simulink model "TestCollecteurAdmissionNew"  (R2024b)
settings: Solver=ode45  StartTime=0.0  StopTime=TempsMaxEvt  MaxStep=0.1  RelTol=1e-9  EnableMultiTasking=on
undefined symbols (not defined in the file): DebitAirEvt, DebitMoteurEvt, ManifoldMassTest, ManifoldPressureTest, ManifoldTemperatureTest, ManifoldTimeTest, Rair, Tamb, TempsEvt, Vcol
settings Model: Creator=a030141  LastModifiedBy=ramse
settings SolverCC: AlgebraicLoopSolver=TrustRegion
settings DataIOCC: LimitDataPoints=on  SaveFormat=Array  SignalLoggingSaveFormat=ModelDataLogs  ReturnWorkspaceOutputs=off  SignalLoggingName=sigsOut
settings OptimizationCC: InitFltsAndDblsToZero=on  LifeSpan=inf
settings DebuggingCC: SaveWithParameterizedLinksMsg=none  UnderspecifiedInitializationDetection=Classic  MergeDetectMultiDrivingBlocksExec=none  SignalResolutionControl=TryResolveAllWithWarning  MultiTaskDSMMsg=warning  MultiTaskCondExecSysMsg=none  FcnCallInpInsideContextMsg=warning  UnconnectedInputMsg=warning  UnconnectedOutputMsg=warning  UnconnectedLineMsg=warning  SFUnexpectedBacktrackingDiag=warning  SFNoUnconditionalDefaultTransitionDiag=warning  SFExecutionAtInitializationDiag=none  ArithmeticOperatorsInVariantConditions=warning
settings HardwareCC: ProdBitPerPointer=32  ProdBitPerSizeT=32  ProdBitPerPtrDiffT=32  ProdLargestAtomicFloat=None  ProdIntDivRoundTo=Undefined  ProdEndianess=Unspecified  ProdWordSize=32  ProdHWDeviceType=32-bit Generic  TargetUnknown=on
settings ModelReferenceCC: PropagateSignalLabelsOutOfModel=off
settings RTWCC: GPUComputeCapability=3.5
settings CodeAppCC: StateflowObjectComments=on
settings GRTTargetCC: TargetFcnLib=ansi_tfl_tmw.mat  TargetLangStandard=C89/C90 (ANSI)  CombineOutputUpdateFcns=off  GRTInterface=on
settings ConfigComp: CovMetricSettings=dw  CovSaveCumulativeToWorkspaceVar=on  CovSaveSingleToWorkspaceVar=on

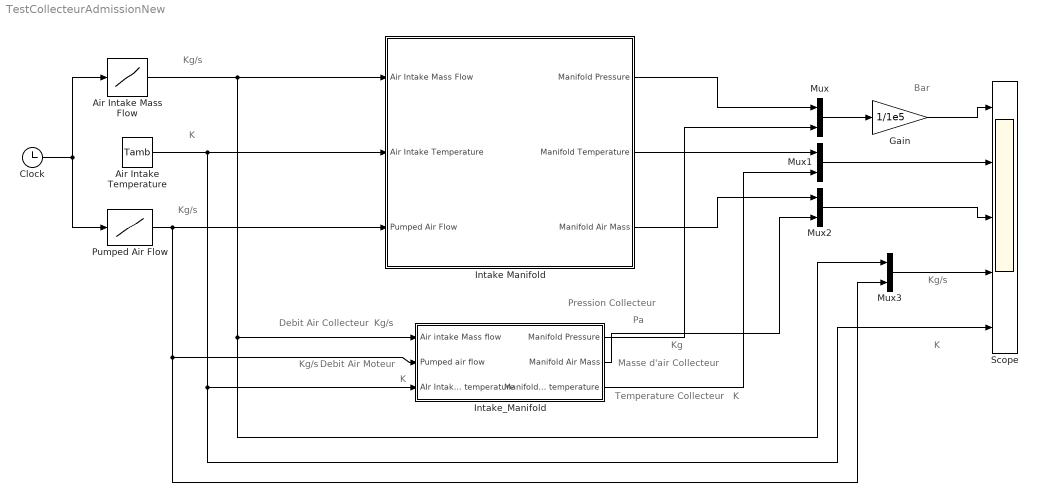
== system TestCollecteurAdmissionNew ==
  note: Debit Air Moteur
  note: Debit Air Collecteur
  note: Temperature Collecteur
  note: Masse d'air Collecteur
  note: Pression Collecteur
  note: Kg/s
  note: Kg/s
  note: Kg/s
  note: Kg/s
  note: K
  note: Kg
  note: K
  note: Pa
  note: K
  note: Bar
  note: Kg/s
  note: K
  Air Intake Mass Flow : Lookup  InputValues=TempsEvt  Table=DebitAirEvt
  Air Intake Temperature : Constant  Value=Tamb
  Clock : Clock
  Gain : Gain  Gain=1/1e5  SaturateOnIntegerOverflow=on  OutDataTypeStr=Inherit: Same as input  ParamDataTypeStr=Inherit: Same as input
  Intake Manifold : Subsystem
  Intake_Manifold : Subsystem
  Mux{,1..3} (4 alike) : Mux  Inputs=2
  Pumped Air Flow : Lookup  InputValues=TempsEvt  Table=DebitMoteurEvt
  Scope : Scope  NumInputPorts=5
  wires:
  Intake_Manifold/1(Manifold Pressure) -> Mux/2
  Air Intake Temperature/1 -> Intake_Manifold/3(AIr Intake temperature), Scope/5, Intake Manifold/2(Air Intake Temperature)
  Intake_Manifold/2(Manifold Air Mass) -> Mux2/2
  Clock/1 -> Pumped Air Flow/1, Air Intake Mass Flow/1
  Air Intake Mass Flow/1 -> Mux3/1, Intake_Manifold/1(Air intake Mass flow), Intake Manifold/1(Air Intake Mass Flow)
  Pumped Air Flow/1 -> Mux3/2, Intake_Manifold/2(Pumped air flow), Intake Manifold/3(Pumped Air Flow)
  Mux/1 -> Gain/1
  Gain/1 -> Scope/1
  Mux1/1 -> Scope/2
  Mux2/1 -> Scope/3
  Mux3/1 -> Scope/4
  Intake Manifold/1(Manifold Pressure) -> Mux/1
  Intake Manifold/2(Manifold Temperature) -> Mux1/1
  Intake Manifold/3(Manifold Air Mass) -> Mux2/1
  Intake_Manifold/3(Manifold temperature) -> Mux1/2

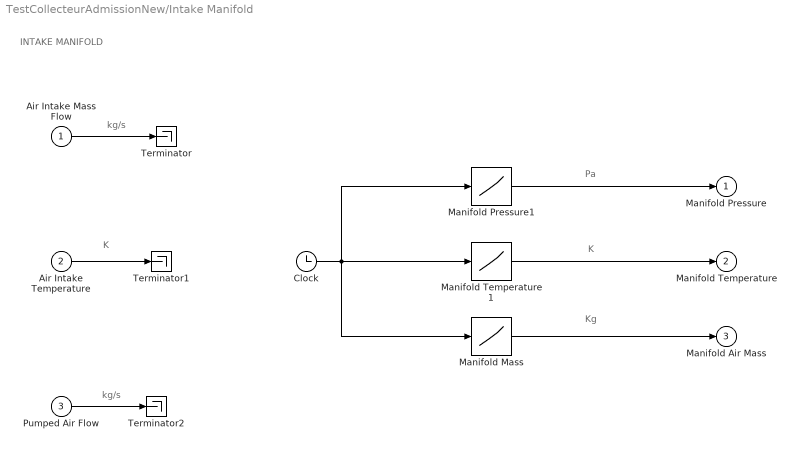
== system TestCollecteurAdmissionNew/Intake Manifold ==
  note: INTAKE MANIFOLD
  note: kg/s
  note: K
  note: kg/s
  note: Kg
  note: K
  note: Pa
  Air Intake Mass Flow : Inport
  Air Intake Temperature : Inport  Port=2
  Pumped Air Flow : Inport  Port=3
  Clock : Clock
  Manifold Mass : Lookup  InputValues=ManifoldTimeTest  Table=ManifoldMassTest
  Manifold Pressure1 : Lookup  InputValues=ManifoldTimeTest  Table=ManifoldPressureTest
  Manifold Temperature1 : Lookup  InputValues=ManifoldTimeTest  Table=ManifoldTemperatureTest
  Terminator : Terminator
  Terminator1 : Terminator
  Terminator2 : Terminator
  Manifold Pressure : Outport
  Manifold Temperature : Outport  Port=2
  Manifold Air Mass : Outport  Port=3
  wires:
  Pumped Air Flow/1 -> Terminator2/1
  Air Intake Mass Flow/1 -> Terminator/1
  Air Intake Temperature/1 -> Terminator1/1
  Manifold Pressure1/1 -> Manifold Pressure/1
  Manifold Temperature1/1 -> Manifold Temperature/1
  Manifold Mass/1 -> Manifold Air Mass/1
  Clock/1 -> Manifold Temperature1/1, Manifold Pressure1/1, Manifold Mass/1

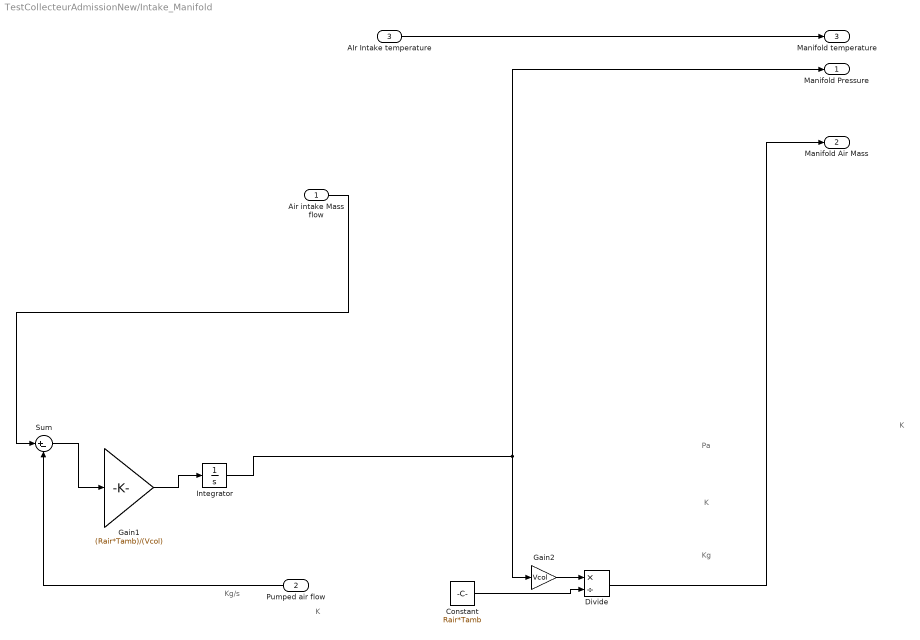
== system TestCollecteurAdmissionNew/Intake_Manifold ==
  note: Kg/s
  note: Kg
  note: K
  note: Pa
  note: K
  note: K
  Air intake Mass flow : Inport
  Pumped air flow : Inport  Port=2
  AIr Intake temperature : Inport  Port=3
  Constant : Constant  Value=Rair*Tamb
  Divide : Product  Inputs=*/
  Gain1 : Gain  Gain=(Rair*Tamb)/(Vcol)
  Gain2 : Gain  Gain=Vcol
  Integrator : Integrator
  Sum : Sum  Inputs=|+-
  Manifold Pressure : Outport
  Manifold Air Mass : Outport  Port=2
  Manifold temperature : Outport  Port=3
  wires:
  Gain2/1 -> Divide/1
  Air intake Mass flow/1 -> Sum/1
  Sum/1 -> Gain1/1
  Divide/1 -> Manifold Air Mass/1
  Gain1/1 -> Integrator/1
  Pumped air flow/1 -> Sum/2
  Constant/1 -> Divide/2
  Integrator/1 -> Manifold Pressure/1, Gain2/1
  AIr Intake temperature/1 -> Manifold temperature/1
